simulink model "Suspension"  (R2021a)
settings: Solver=VariableStepAuto  StartTime=0.0  StopTime=50  RelTol=1e-3
undefined symbols (not defined in the file): Cs, Ct, Ks, Kt, ms, mu, xf
libraries: simulink x1
settings Model: Creator=90554  LastModifiedBy=90554

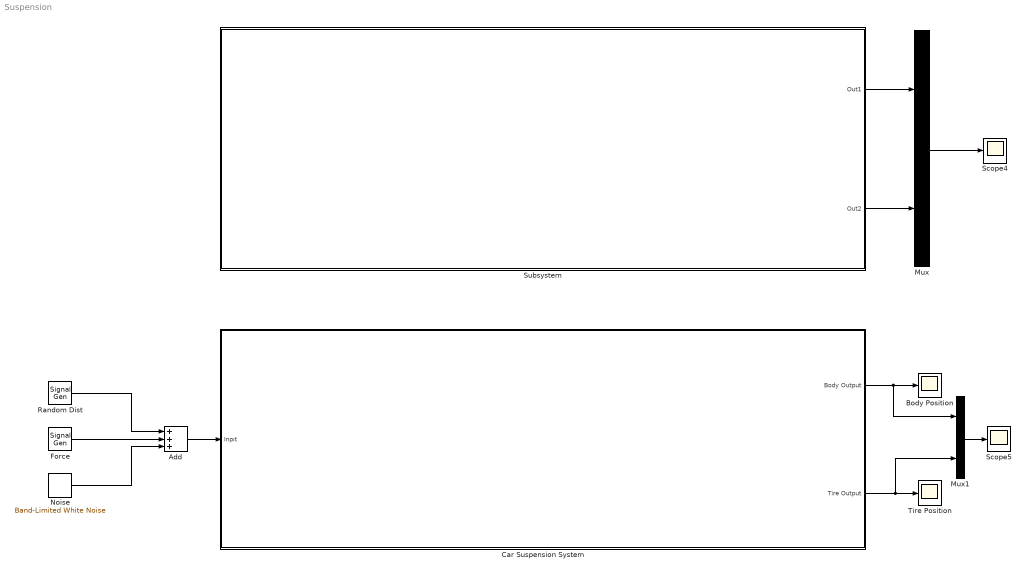
== system Suspension ==
  Add : Sum  Inputs=+++
  Body Position : Scope
  Car Suspension System : Subsystem
      mask Display: image(imread('A-quarter-car-model-of-suspension-system.png'))
  Force : SignalGenerator  WaveForm=square  Amplitude=-1000  Frequency=0.01
  Mux : Mux  Inputs=2
  Mux1 : Mux  Inputs=2
  Noise : simulink/Sources/Band-Limited White Noise  Cov=[0.1]  Ts=0.1  seed=[23341]
  Random Dist : SignalGenerator  WaveForm=random  Amplitude=25  Units=rad/sec
  Scope4 : Scope
  Scope5 : Scope
  Subsystem : Subsystem
      mask Display: image(imread('accord_vars.jpg'))
  Tire Position : Scope
  wires:
  Mux/1 -> Scope4/1
  Force/1 -> Add/2
  Random Dist/1 -> Add/1
  Noise/1 -> Add/3
  Add/1 -> Car Suspension System/1(Inpıt)
  Car Suspension System/1(Body Output) -> Body Position/1, Mux1/1
  Car Suspension System/2(Tire Output) -> Tire Position/1, Mux1/2
  Mux1/1 -> Scope5/1
  Subsystem/1(Out1) -> Mux/1
  Subsystem/2(Out2) -> Mux/2

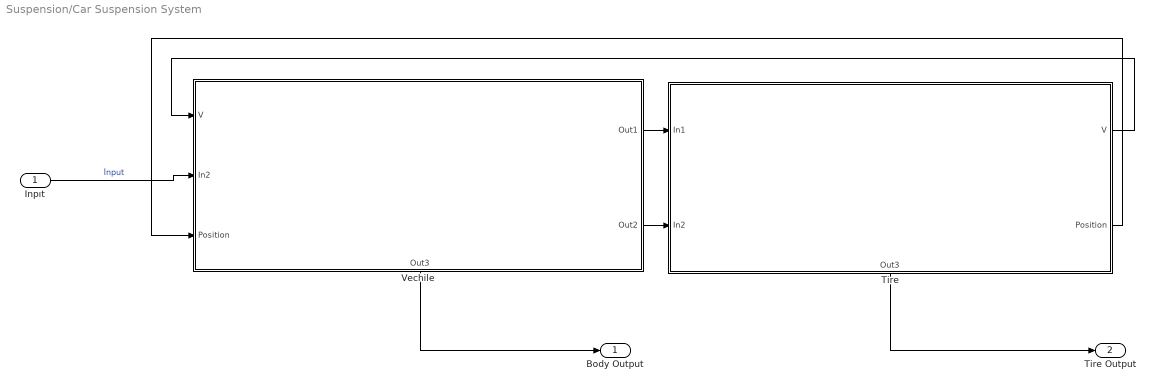
== system Suspension/Car Suspension System ==
  Inpıt : Inport
  Tire : Subsystem
      settings: PortSchema="{\"entries\":[{\"content\":{\"sides\":[{\"content\":{\"connectorIds\":[\"In1\",\"In2\"]},\"type\":\"ConnectorPlacement.EquallySpacedRectSide\",\"uuid\":\"02e87868-6275-4d3c-ac43-40359a3a8891\"},{\"content\":{\"connectorIds\":[\"Out1\",\"Out2\"],\"side\":\"RIGHT\"},\"type\":\"ConnectorPlacement.EquallySpacedRectSide\",\"uuid\":\"93b2f076-b23b-4d7d-991d-853ba946847a\"},{\"content\":{\"connectorIds\":[],\"side\":\"TOP\"},\"type\":\"ConnectorPlacement.EquallySpacedRectSide\",\"uuid\":\"73c7a1ee-55a8-412d-8814-a53f381b6b5c\"},{\"content\":{\"connectorIds\":[\"Out3\"],\"side\":\"BOTTOM\"},\"type\":\"ConnectorPlacement.EquallySpacedRectSide\",\"uuid\":\"0b1c754c-f6ba-44db-8ff2-50875a392fde\"}]},\"type\":\"ConnectorPlacement.EquallySpacedConnector\",\"uuid\":\"a1b90636-88af-4198-948a-e6671dff3ad8\"}],\"packageUris\":[\"http://schema.mathworks.com/mf0/Connector/R2020b\"],\"version\":\"1.0\"}"
  Vechile : Subsystem
      settings: PortSchema="{\"entries\":[{\"content\":{\"sides\":[{\"content\":{\"connectorIds\":[\"In1\",\"In2\",\"In3\"]},\"type\":\"ConnectorPlacement.EquallySpacedRectSide\",\"uuid\":\"f42c1fa4-fba4-46c9-8960-6c9b44803588\"},{\"content\":{\"connectorIds\":[\"Out1\",\"Out2\"],\"side\":\"RIGHT\"},\"type\":\"ConnectorPlacement.EquallySpacedRectSide\",\"uuid\":\"574e747f-4e5b-453e-a072-2b77a5cfabcf\"},{\"content\":{\"connectorIds\":[],\"side\":\"TOP\"},\"type\":\"ConnectorPlacement.EquallySpacedRectSide\",\"uuid\":\"0ac87736-0a65-4cd4-81d6-fe4dd954ca2d\"},{\"content\":{\"connectorIds\":[\"Out3\"],\"side\":\"BOTTOM\"},\"type\":\"ConnectorPlacement.EquallySpacedRectSide\",\"uuid\":\"a6aa5f83-93fe-450c-b61a-5bd7a54be2e2\"}]},\"type\":\"ConnectorPlacement.EquallySpacedConnector\",\"uuid\":\"07668f95-5f8b-4280-89c2-4867d000697b\"}],\"packageUris\":[\"http://schema.mathworks.com/mf0/Connector/R2020b\"],\"version\":\"1.0\"}"
  Body Output : Outport
  Tire Output : Outport  Port=2
  wires:
  Vechile/3(Out3) -> Body Output/1
  Tire/2(Position) -> Vechile/3(Position)
  Tire/1(V) -> Vechile/1(V)
  Tire/3(Out3) -> Tire Output/1
  Vechile/1(Out1) -> Tire/1(In1)
  Vechile/2(Out2) -> Tire/2(In2)
  Inpıt/1 -> Vechile/2(In2)  "İnput"

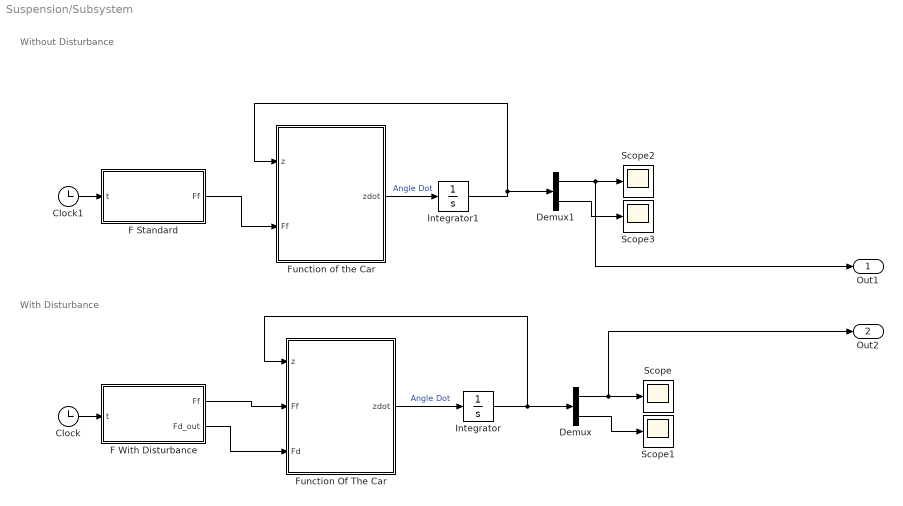
== system Suspension/Subsystem ==
  note: With Disturbance
  note: Without Disturbance
  Clock : Clock
  Clock1 : Clock
  Demux : Demux  Outputs=2
  Demux1 : Demux  Outputs=2
  F Standard : MATLAB Function  TreatAsAtomicUnit=on
  "F With Disturbance " : MATLAB Function  TreatAsAtomicUnit=on
  Function Of The Car : MATLAB Function  TreatAsAtomicUnit=on
  "Function of the Car " : MATLAB Function  TreatAsAtomicUnit=on
  Integrator : Integrator  InitialCondition=[0;0]
  Integrator1 : Integrator  InitialCondition=[0;0]
  Scope{,1..3} (4 alike) : Scope
  Out1 : Outport
  Out2 : Outport  Port=2
  wires:
  "F With Disturbance "/2(Fd_out) -> Function Of The Car/3(Fd)
  Clock/1 -> "F With Disturbance "/1(t)
  Integrator1/1 -> Demux1/1, "Function of the Car "/1(z)
  Integrator/1 -> Demux/1, Function Of The Car/1(z)
  Demux/2 -> Scope1/1
  Demux/1 -> Out2/1, Scope/1
  "F With Disturbance "/1(Ff) -> Function Of The Car/2(Ff)
  Demux1/1 -> Out1/1, Scope2/1
  Demux1/2 -> Scope3/1
  Function Of The Car/1(zdot) -> Integrator/1  "Angle Dot"
  "Function of the Car "/1(zdot) -> Integrator1/1  "Angle Dot"
  F Standard/1(Ff) -> "Function of the Car "/2(Ff)
  Clock1/1 -> F Standard/1(t)

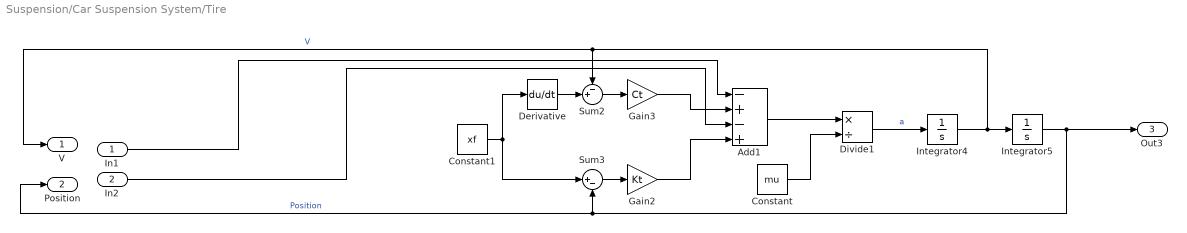
== system Suspension/Car Suspension System/Tire ==
  In1 : Inport
  In2 : Inport  Port=2
  Add1 : Sum  Inputs=-+-+
  Constant : Constant  Value=mu
  Constant1 : Constant  Value=xf
  Derivative : Derivative
  Divide1 : Product  Inputs=*/
  Gain2 : Gain  Gain=Kt
  Gain3 : Gain  Gain=Ct
  Integrator4 : Integrator
  Integrator5 : Integrator
  Sum2 : Sum  Inputs=-+|
  Sum3 : Sum  Inputs=|+-
  V : Outport
  Position : Outport  Port=2
  Out3 : Outport  Port=3
  wires:
  Integrator4/1 -> V/1, Sum2/1, Integrator5/1  "V"
  Add1/1 -> Divide1/1
  Derivative/1 -> Sum2/2
  Constant/1 -> Divide1/2
  Constant1/1 -> Derivative/1, Sum3/1
  In1/1 -> Add1/1
  Divide1/1 -> Integrator4/1  "a"
  Sum3/1 -> Gain2/1
  Sum2/1 -> Gain3/1
  Integrator5/1 -> Out3/1, Position/1, Sum3/2  "Position"
  Gain3/1 -> Add1/2
  Gain2/1 -> Add1/4
  In2/1 -> Add1/3

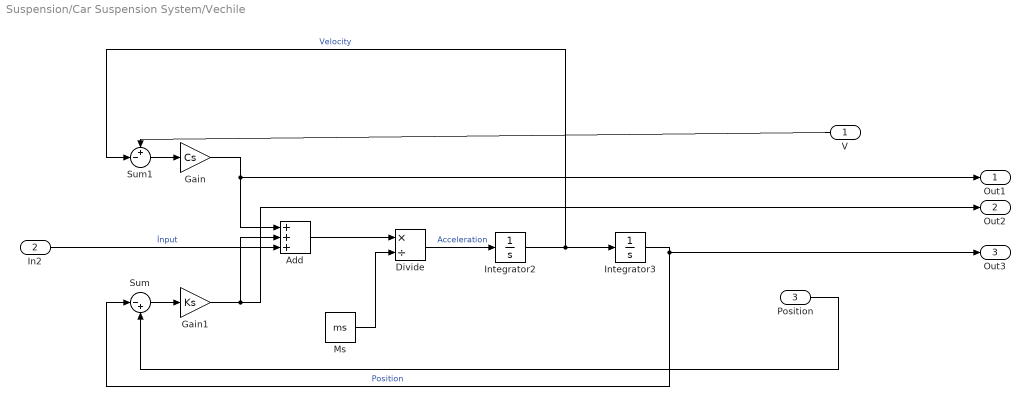
== system Suspension/Car Suspension System/Vechile ==
  V : Inport
  In2 : Inport  Port=2
  Position : Inport  Port=3
  Add : Sum  Inputs=+++
  Divide : Product  Inputs=*/
  Gain : Gain  Gain=Cs
  Gain1 : Gain  Gain=Ks
  Integrator2 : Integrator
  Integrator3 : Integrator
  Ms : Constant  Value=ms
  Sum : Sum  Inputs=|-+
  Sum1 : Sum  Inputs=+-|
  Out1 : Outport
  Out2 : Outport  Port=2
  Out3 : Outport  Port=3
  wires:
  Integrator3/1 -> Out3/1, Sum/1  "Position"
  Sum1/1 -> Gain/1
  Integrator2/1 -> Sum1/2, Integrator3/1  "Velocity"
  Gain/1 -> Out1/1, Add/1
  Add/1 -> Divide/1
  Sum/1 -> Gain1/1
  Gain1/1 -> Out2/1, Add/2
  Divide/1 -> Integrator2/1  "Acceleration"
  Ms/1 -> Divide/2
  In2/1 -> Add/3  "İnput"
  Position/1 -> Sum/2
  V/1 -> Sum1/1

== matlab function Suspension/Subsystem/F With Disturbance  ==
  data: t input; Ff output; Fd_out output
function  [Ff, Fd_out]= fcn(t)

ff_int = 0;

t_mod = mod(t,10);

if t_mod<3
    
    ff_int = 1500;
    
end

if t_mod>=3 && t_mod<5
    
    ff_int=300;

end

if t_mod>=5 && t_mod<8
    
    ff_int=2000;

end

if t_mod>=8 && t_mod<10
    
    ff_int=850;

end

%% Disturbance
f = 0.1;

Fd= 0.00009*sin(2*pi*f*t);
Fd_Dot = 0.00009*(2*pi*t)*cos(2*pi*f*t);

%Out
Ff = ff_int;
Fd_out = [Fd; Fd_Dot];
end

== matlab function Suspension/Subsystem/Function Of The Car ==
  data: z input; zdot output; Ff input; Fd input
function zdot = fcn(z,Ff,Fd)

% theta = z(1,1);
% theta_dot = z(2,1);

Lb = 1; %Arka uzunluk m çinsinde
Lf =1; %Ön uzunluk
Lh = 0.3; %Aracın yerden yüksekliği
mcar = 1500; %Kütle


Kyf =25000;
Kyb = 25000;
Cyf =1000;
Cyb =1000;


%%
Icar = 1/12*mcar*((Lb+Lf)/2)^2;

Kt = Lf*Kyf +Lb*Kyb;
Ct = Lf*Cyf+Lb*Cyb;

%%
A =[0,1;-Kt/Icar, -Ct/Icar];
B =[0;Lh/Icar];
D = [ 0 0; Kt/mcar Ct/mcar];

%%Output
zdot = A*z +B*Ff + D*Fd;

% y1 = theta*Lf; %Deflection 
% y2 = -theta*Lf; %Deflection
% 
% fyf = theta*Lf*Kyf + theta_dot*Lf*Cyf; % Frontal Force
% fyb =  -(theta*Lb*Kyb+ theta_dot*Lb*Cyb); %Back Force
% 
% 
% fyf_k = theta*Lf*Kyf; %Check the our suspension K, This value is factory data of spring constant.
% fyf_b = -theta*Lb*Kyb;
% 
% 
% fyf_c = theta_dot*Lf*Cyf; % Check the our suspension C, This value is factory data of C constant.
% fyb_c = -theta_dot*Lb*Cyb;





end

== matlab function Suspension/Subsystem/F Standard ==
  data: t input; Ff output
function  Ff= fcn(t)

ff_int = 0;

t_mod = mod(t,10);

if t_mod<3
    
    ff_int = 1500;
    
end

if t_mod>=3 && t_mod<5
    
    ff_int=300;

end

if t_mod>=5 && t_mod<8
    
    ff_int=2000;

end

if t_mod>=8 && t_mod<10
    
    ff_int=850;

end


%Out
Ff = ff_int;

end

== matlab function Suspension/Subsystem/Function of the Car  ==
  data: z input; zdot output; Ff input
function zdot = fcn(z,Ff)

% theta = z(1,1);
% theta_dot = z(2,1);

Lb = 1; %Arka uzunluk m çinsinde
Lf =1; %Ön uzunluk
Lh = 0.3; %Aracın yerden yüksekliği
mcar = 1500; %Kütle


Kyf =25000;
Kyb = 25000;
Cyf =1000;
Cyb =1000;


%%
Icar = 1/12*mcar*((Lb+Lf)/2)^2;

Kt = Lf*Kyf +Lb*Kyb;
Ct = Lf*Cyf+Lb*Cyb;

%%
A =[0,1;-Kt/Icar, -Ct/Icar];
B =[0;Lh/Icar];


%%Output
zdot = A*z +B*Ff;

% y1 = theta*Lf; %Deflection 
% y2 = -theta*Lf; %Deflection
% 
% fyf = theta*Lf*Kyf + theta_dot*Lf*Cyf; % Frontal Force
% fyb =  -(theta*Lb*Kyb+ theta_dot*Lb*Cyb); %Back Force
% 
% 
% fyf_k = theta*Lf*Kyf; %Check the our suspension K, This value is factory data of spring constant.
% fyf_b = -theta*Lb*Kyb;
% 
% 
% fyf_c = theta_dot*Lf*Cyf; % Check the our suspension C, This value is factory data of C constant.
% fyb_c = -theta_dot*Lb*Cyb;





end
